simulink model "Lab01P4"  (Simulink 7.1)
settings: Solver=ode45  StartTime=0.0  StopTime=10.0  RelTol=1e-3
settings Model: Creator=ALUNO  LastModifiedBy=ALUNO

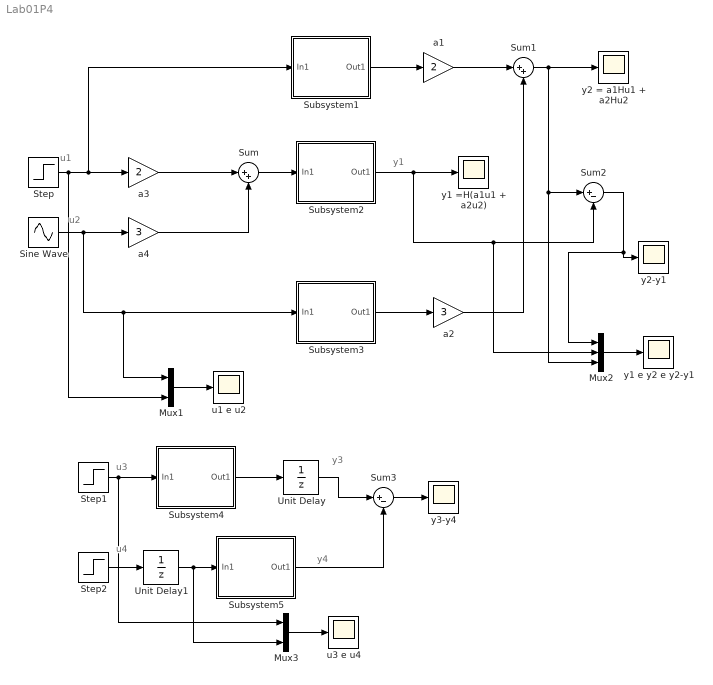
== system Lab01P4 ==
  note: y3
  note: y4
  note: u4
  note: u3
  note: y1
  note: u1
  note: u2
  Mux1 : Mux  Inputs=2
  Mux2 : Mux  Inputs=3
  Mux3 : Mux  Inputs=2
  Sine Wave : Sin  SampleTime=0
  Step : Step  Time=0  SampleTime=0
  Step1 : Step  Time=0  SampleTime=0
  Step2 : Step  Time=0  SampleTime=0
  Subsystem1 : Subsystem
      mask Display: disp('Planta P4')
  Subsystem2 : Subsystem
      mask Display: disp('Planta P4')
  Subsystem3 : Subsystem
      mask Display: disp('Planta P4')
  Subsystem4 : Subsystem
      mask Display: disp('Planta P4')
  Subsystem5 : Subsystem
      mask Display: disp('Planta P4')
  Sum : Sum  Inputs=|++  OutDataType=sfix(16)  OutScaling=2^0
  Sum1 : Sum  Inputs=|++  OutDataType=sfix(16)  OutScaling=2^0
  Sum2 : Sum  Inputs=|+-  OutDataType=sfix(16)  OutScaling=2^0
  Sum3 : Sum  Inputs=|+-  OutDataType=sfix(16)  OutScaling=2^0
  Unit Delay : UnitDelay
  Unit Delay1 : UnitDelay
  a1 : Gain  Gain=2  ParameterDataType=sfix(16)  ParameterScaling=2^0  OutDataType=sfix(16)  OutScaling=2^0
  a2 : Gain  Gain=3  ParameterDataType=sfix(16)  ParameterScaling=2^0  OutDataType=sfix(16)  OutScaling=2^0
  a3 : Gain  Gain=2  ParameterDataType=sfix(16)  ParameterScaling=2^0  OutDataType=sfix(16)  OutScaling=2^0
  a4 : Gain  Gain=3  ParameterDataType=sfix(16)  ParameterScaling=2^0  OutDataType=sfix(16)  OutScaling=2^0
  u1 e u2 : Scope
      settings: SaveName=ScopeData6
  u3 e u4 : Scope
      settings: SaveName=ScopeData3
  y1 =H(a1u1 + a2u2) : Scope
  y1 e y2 e y2-y1 : Scope
      settings: SaveName=ScopeData5
  y2 = a1Hu1 + a2Hu2 : Scope
  y2-y1 : Scope
      settings: SaveName=ScopeData2
  y3-y4 : Scope
      settings: SaveName=ScopeData7
  wires:
  Step/1 -> a3/1, Subsystem1/1(In1), Mux1/2
  a3/1 -> Sum/1
  Sine Wave/1 -> a4/1, Mux1/1, Subsystem3/1(In1)
  a4/1 -> Sum/2
  Sum/1 -> Subsystem2/1(In1)
  Subsystem1/1(Out1) -> a1/1
  Subsystem2/1(Out1) -> y1 =H(a1u1 + a2u2)/1, Sum2/2, Mux2/2
  a1/1 -> Sum1/1
  Subsystem3/1(Out1) -> a2/1
  a2/1 -> Sum1/2
  Sum1/1 -> y2 = a1Hu1 + a2Hu2/1, Sum2/1, Mux2/3
  Sum2/1 -> y2-y1/1, Mux2/1
  Mux1/1 -> u1 e u2/1
  Mux2/1 -> y1 e y2 e y2-y1/1
  Step1/1 -> Mux3/1, Subsystem4/1(In1)
  Subsystem4/1(Out1) -> Unit Delay/1
  Step2/1 -> Unit Delay1/1
  Unit Delay1/1 -> Subsystem5/1(In1), Mux3/2
  Unit Delay/1 -> Sum3/1
  Subsystem5/1(Out1) -> Sum3/2
  Sum3/1 -> y3-y4/1
  Mux3/1 -> u3 e u4/1

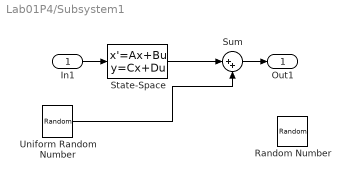
== system Lab01P4/Subsystem1 ==
  In1 : Inport  OutDataType=sfix(16)  OutScaling=2^0
  Random Number : RandomNumber  Variance=0.25  SampleTime=0
  State-Space : StateSpace  A=[-1 -2;1 0]  B=[1; 0]  C="[0  2]"  D=0
  Sum : Sum  Inputs=|++  OutDataType=sfix(16)  OutScaling=2^0
  Uniform Random Number : UniformRandomNumber  Minimum=-0.25  Maximum=0.25  SampleTime=0
  Out1 : Outport  OutDataType=sfix(16)  OutScaling=2^0
  wires:
  State-Space/1 -> Sum/1
  In1/1 -> State-Space/1
  Sum/1 -> Out1/1
  Uniform Random Number/1 -> Sum/2

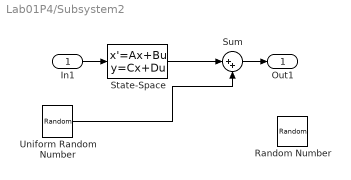
== system Lab01P4/Subsystem2 ==
  In1 : Inport  OutDataType=sfix(16)  OutScaling=2^0
  Random Number : RandomNumber  Variance=0.25  SampleTime=0
  State-Space : StateSpace  A=[-1 -2;1 0]  B=[1; 0]  C="[0  2]"  D=0
  Sum : Sum  Inputs=|++  OutDataType=sfix(16)  OutScaling=2^0
  Uniform Random Number : UniformRandomNumber  Minimum=-0.25  Maximum=0.25  SampleTime=0
  Out1 : Outport  OutDataType=sfix(16)  OutScaling=2^0
  wires:
  State-Space/1 -> Sum/1
  In1/1 -> State-Space/1
  Sum/1 -> Out1/1
  Uniform Random Number/1 -> Sum/2

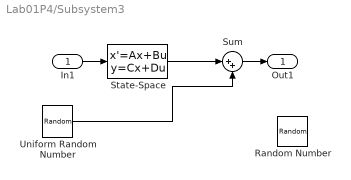
== system Lab01P4/Subsystem3 ==
  In1 : Inport  OutDataType=sfix(16)  OutScaling=2^0
  Random Number : RandomNumber  Variance=0.25  SampleTime=0
  State-Space : StateSpace  A=[-1 -2;1 0]  B=[1; 0]  C="[0  2]"  D=0
  Sum : Sum  Inputs=|++  OutDataType=sfix(16)  OutScaling=2^0
  Uniform Random Number : UniformRandomNumber  Minimum=-0.25  Maximum=0.25  SampleTime=0
  Out1 : Outport  OutDataType=sfix(16)  OutScaling=2^0
  wires:
  State-Space/1 -> Sum/1
  In1/1 -> State-Space/1
  Sum/1 -> Out1/1
  Uniform Random Number/1 -> Sum/2

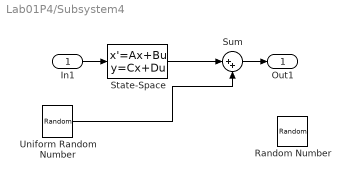
== system Lab01P4/Subsystem4 ==
  In1 : Inport  OutDataType=sfix(16)  OutScaling=2^0
  Random Number : RandomNumber  Variance=0.25  SampleTime=0
  State-Space : StateSpace  A=[-1 -2;1 0]  B=[1; 0]  C="[0  2]"  D=0
  Sum : Sum  Inputs=|++  OutDataType=sfix(16)  OutScaling=2^0
  Uniform Random Number : UniformRandomNumber  Minimum=-0.25  Maximum=0.25  SampleTime=0
  Out1 : Outport  OutDataType=sfix(16)  OutScaling=2^0
  wires:
  State-Space/1 -> Sum/1
  In1/1 -> State-Space/1
  Sum/1 -> Out1/1
  Uniform Random Number/1 -> Sum/2

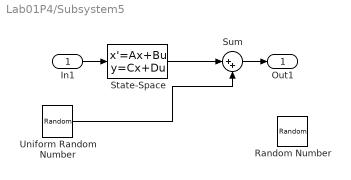
== system Lab01P4/Subsystem5 ==
  In1 : Inport  OutDataType=sfix(16)  OutScaling=2^0
  Random Number : RandomNumber  Variance=0.25  SampleTime=0
  State-Space : StateSpace  A=[-1 -2;1 0]  B=[1; 0]  C="[0  2]"  D=0
  Sum : Sum  Inputs=|++  OutDataType=sfix(16)  OutScaling=2^0
  Uniform Random Number : UniformRandomNumber  Minimum=-0.25  Maximum=0.25  SampleTime=0
  Out1 : Outport  OutDataType=sfix(16)  OutScaling=2^0
  wires:
  State-Space/1 -> Sum/1
  In1/1 -> State-Space/1
  Sum/1 -> Out1/1
  Uniform Random Number/1 -> Sum/2
